simulink model "designSmcLq2009b"  (Simulink 7.4)
settings: Solver=ode3  StartTime=0.0  StopTime=10  FixedStep=Ts  RelTol=1e-3
values from neighbouring files (symbols this model uses):
  A = [0.0 1.0 0.0 0.0 ... (first row only)    [designSmcLq_sim.m]
  amp = 1    [designSmcLq_sim.m]
  B = [0.0 ... (first row only)    [designSmcLq_sim.m]
  eta = 1e-1    (= 0.1)    [designSmcLq_sim.m]
  Klq = lqr(A,B,Q,R)    [designSmcLq_sim.m]
  Ksmcl = inv(S*B)*S*A    [designSmcLq_sim.m]
  Ksmcnl = 4    [designSmcLq_sim.m]
  S = lqr(A,B,Q,R)    [designSmcLq_sim.m]
  x0 = [0 ... (first row only)    [designSmcLq_sim.m]
settings Model: Creator=Yu  LastModifiedBy=Yu
settings DataIOCC: SaveFormat=StructureWithTime
settings OptimizationCC: ExpressionDepthLimit=128
settings DebuggingCC: UnderspecifiedInitializationDetection=Simplified  MergeDetectMultiDrivingBlocksExec=error  SolverPrmCheckMsg=none  FcnCallInpInsideContextMsg=Enable All  StateNameClashWarn=none  StrictBusMsg=ErrorLevel1
settings HardwareCC: ProdIntDivRoundTo=Zero  ProdEndianess=LittleEndian  ProdHWDeviceType=Specified
settings CodeAppCC: CustomSymbolStrType=$N$R$M_T
settings GRTTargetCC: TargetFunctionLibrary=C89/C90 (ANSI)  GeneratePreprocessorConditionals=Use local settings

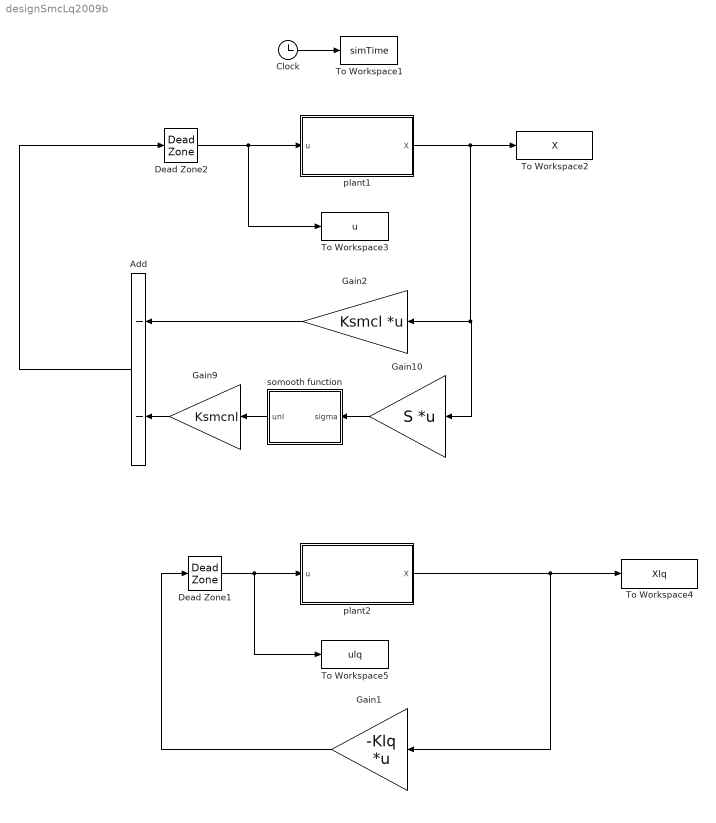
== system designSmcLq2009b ==
  Add : Sum  Inputs=--
  Clock : Clock
  Dead Zone1 : DeadZone  LowerValue=-amp  UpperValue=amp  SaturateOnIntegerOverflow=on
  Dead Zone2 : DeadZone  LowerValue=-amp  UpperValue=amp  SaturateOnIntegerOverflow=on
  Gain1 : Gain  Gain=-Klq  Multiplication=Matrix(K*u)
  Gain10 : Gain  Gain=S  Multiplication=Matrix(K*u)
  Gain2 : Gain  Gain=Ksmcl  Multiplication=Matrix(K*u)
  Gain9 : Gain  Gain=Ksmcnl
  To Workspace1 : ToWorkspace  VariableName=simTime  SampleTime=-1
  To Workspace2 : ToWorkspace  VariableName=X  SampleTime=-1
  To Workspace3 : ToWorkspace  VariableName=u  SampleTime=-1
  To Workspace4 : ToWorkspace  VariableName=Xlq  SampleTime=-1
  To Workspace5 : ToWorkspace  VariableName=ulq  SampleTime=-1
  plant1 : Subsystem
  plant2 : Subsystem
  somooth function : Subsystem
  wires:
  Clock/1 -> To Workspace1/1
  somooth function/1(unl) -> Gain9/1
  Gain10/1 -> somooth function/1(sigma)
  plant1/1(X) -> Gain10/1, Gain2/1, To Workspace2/1
  Gain9/1 -> Add/2
  Gain2/1 -> Add/1
  Add/1 -> Dead Zone2/1
  plant2/1(X) -> Gain1/1, To Workspace4/1
  Gain1/1 -> Dead Zone1/1
  Dead Zone2/1 -> To Workspace3/1, plant1/1(u)
  Dead Zone1/1 -> To Workspace5/1, plant2/1(u)

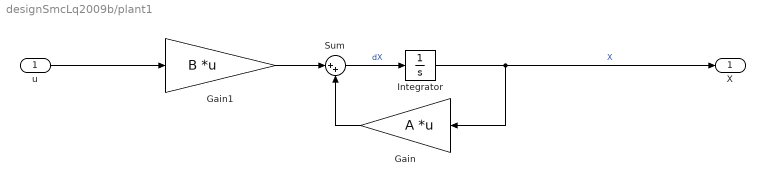
== system designSmcLq2009b/plant1 ==
  u : Inport
  Gain : Gain  Gain=A  Multiplication=Matrix(K*u)
  Gain1 : Gain  Gain=B  Multiplication=Matrix(K*u)
  Integrator : Integrator  InitialCondition=x0
  Sum : Sum  Inputs=|++
  X : Outport
  wires:
  Gain/1 -> Sum/2
  Integrator/1 -> X/1, Gain/1  "X"
  Sum/1 -> Integrator/1  "dX"
  Gain1/1 -> Sum/1
  u/1 -> Gain1/1

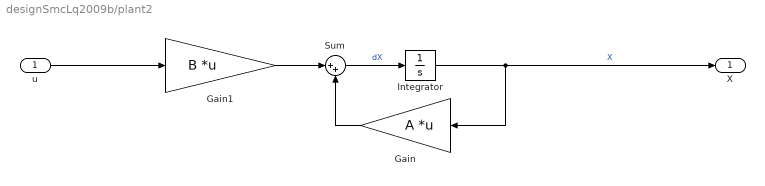
== system designSmcLq2009b/plant2 ==
  u : Inport
  Gain : Gain  Gain=A  Multiplication=Matrix(K*u)
  Gain1 : Gain  Gain=B  Multiplication=Matrix(K*u)
  Integrator : Integrator  InitialCondition=x0
  Sum : Sum  Inputs=|++
  X : Outport
  wires:
  Gain/1 -> Sum/2
  Integrator/1 -> X/1, Gain/1  "X"
  Sum/1 -> Integrator/1  "dX"
  Gain1/1 -> Sum/1
  u/1 -> Gain1/1

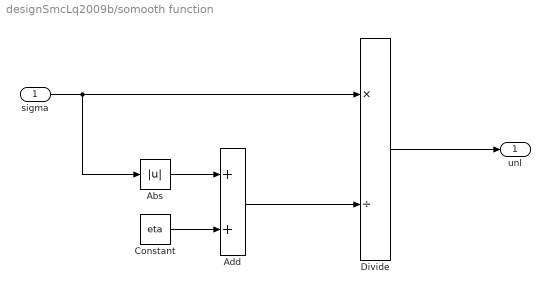
== system designSmcLq2009b/somooth function ==
  sigma : Inport
  Abs : Abs
  Add : Sum
  Constant : Constant  Value=eta
  Divide : Product  Inputs=*/
  unl : Outport
  wires:
  Abs/1 -> Add/1
  Constant/1 -> Add/2
  sigma/1 -> Abs/1, Divide/1
  Add/1 -> Divide/2
  Divide/1 -> unl/1
